simulink model "PHVS_WithACC"  (R2019b)
settings: Solver=VariableStepAuto  StartTime=0.0  StopTime=1.5  FixedStep=0.00001  MinStep=0.0001  RelTol=1e-3
libraries: fl_lib x25, nesl_utility x11, cstblocks x1
settings Model: Creator=se108102  LastModifiedBy=se108102
settings SFSimCC: CustomCodeUndefinedFunction=UseInterfaceOnly

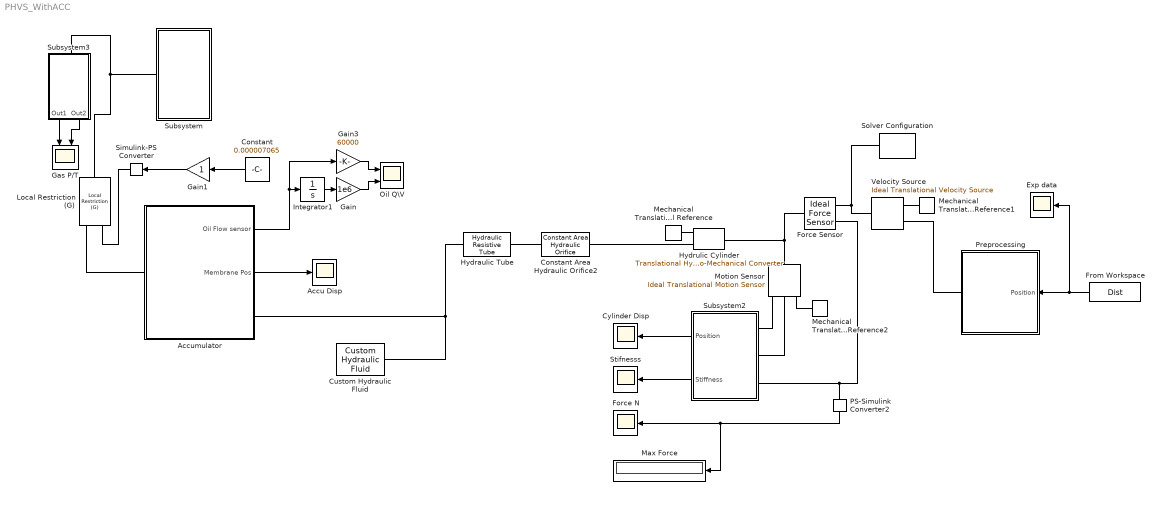
== system PHVS_WithACC ==
  " Force Sensor" : fl_lib/Mechanical/Mechanical Sensors/Ideal Force Sensor
  "Accu Disp " : Scope
  Accumulator : Subsystem
      mask Display: image('ACC.JPG'); % Use "Edit Image" on toolstrip to change.
  Constant : Constant  Value=0.000007065
  Constant Area Hydraulic Orifice2 : fl_lib/Hydraulic/Hydraulic Elements/Constant Area Hydraulic Orifice  area=19.62 mm^2  C_d=.41  lam_spec=1  B_lam=0.999  Re_cr=12  q_specify=off  q_priority=None  q=0.001 m^3/s  q_nominal_specify=off  q_nominal_unit=m^3/s  q_nominal_value=1  p_specify=on  p_priority=None  p=0 Pa  p_nominal_specify=off  p_nominal_unit=Pa  p_nominal_value=1
      settings: SourceProductName=Simscape  SourceProductBaseCode=SS  InternalSimscapePortConfiguration="{\"Bottom\":[],\"Left\":[{\"id\":\"A\",\"label\":\"A\",\"type\":\"foundation.hydraulic.hydraulic\"}],\"Right\":[{\"id\":\"B\",\"label\":\"B\",\"type\":\"foundation.hydraulic.hydraulic\"}],\"Top\":[]}"
  Custom Hydraulic Fluid : fl_lib/Hydraulic/Hydraulic Utilities/Custom Hydraulic Fluid  density=850 kg/m^3  viscosity_kin=18e-6 m^2/s  bulk=0.8e9 Pa  alpha=0.005  range_error=2
      settings: SourceProductName=Simscape  SourceProductBaseCode=SS  InternalSimscapePortConfiguration="{\"Bottom\":[],\"Left\":[],\"Right\":[{\"id\":\"G\",\"label\":\"\",\"type\":\"foundation.hydraulic.hydraulic\"}],\"Top\":[]}"
  Cylinder Disp : Scope
  Exp data : Scope
  Force N : Scope
  From Workspace : FromWorkspace  VariableName=Dist
  Gain : Gain  Gain=1e6
  Gain1 : Gain
  Gain3 : Gain  Gain=60000
  Gas P/T : Scope  NumInputPorts=2
  Hydraulic Tube : fl_lib/Hydraulic/Hydraulic Elements/Hydraulic Resistive Tube  cs_type=1  d_in=10 mm  area=1e-4 m^2  D_h=1.12e-2 m  s_factor=64  length=10 cm  length_ad=1 m  roughness=15e-6 m  Re_lam=2000  Re_turb=4000  q_specify=off  q_priority=None  q=0.001 m^3/s  q_nominal_specify=off  q_nominal_unit=m^3/s  q_nominal_value=1  p_specify=off  p_priority=None  p=0 Pa  p_nominal_specify=off  p_nominal_unit=Pa  p_nominal_value=1
      settings: SourceProductName=Simscape  SourceProductBaseCode=SS  InternalSimscapePortConfiguration="{\"Bottom\":[],\"Left\":[{\"id\":\"A\",\"label\":\"A\",\"type\":\"foundation.hydraulic.hydraulic\"}],\"Right\":[{\"id\":\"B\",\"label\":\"B\",\"type\":\"foundation.hydraulic.hydraulic\"}],\"Top\":[]}"
  Hydrulic Cylinder : fl_lib/Hydraulic/Hydraulic Elements/Translational Hydro-Mechanical Converter  area=12.56 cm^2  or=1  compressibility=0  init_pos=0 m  V_dead=1e-4 m^3  k_sh=1.4  initial_pressure=0 Pa
      settings: SourceProductName=Simscape  SourceProductBaseCode=SS  InternalSimscapePortConfiguration="{\"Bottom\":[],\"Left\":[{\"id\":\"C\",\"label\":\"C\",\"type\":\"foundation.mechanical.translational.translational\"},{\"id\":\"A\",\"label\":\"A\",\"type\":\"foundation.hydraulic.hydraulic\"}],\"Right\":[{\"id\":\"R\",\"label\":\"R\",\"type\":\"foundation.mechanical.translational.translational\"}],\"Top\":[]}"
  Integrator1 : Integrator
  Local Restriction (G) : fl_lib/Gas/Elements/Local Restriction (G)  restriction_type=foundation.enum.restriction_type.variable  restriction_area=1e-3 m^2  min_area=1e-10 m^2  max_area=0.005 m^2  area=0.01 m^2  Cd=0.02  B_lam=0.999
      settings: SourceProductName=Simscape  SourceProductBaseCode=SS  InternalSimscapePortConfiguration="{\"Bottom\":[],\"Left\":[{\"id\":\"A\",\"label\":\"A\",\"type\":\"foundation.gas.gas\"},{\"id\":\"area_in\",\"label\":\"AR\",\"type\":\"input\"}],\"Right\":[{\"id\":\"B\",\"label\":\"B\",\"type\":\"foundation.gas.gas\"}],\"Top\":[]}"
  Max Force : Display
  Mechanical Translational Reference : fl_lib/Mechanical/Translational Elements/Mechanical Translational Reference
  Mechanical Translational Reference1 : fl_lib/Mechanical/Translational Elements/Mechanical Translational Reference
  Mechanical Translational Reference2 : fl_lib/Mechanical/Translational Elements/Mechanical Translational Reference
  Motion Sensor : fl_lib/Mechanical/Mechanical Sensors/Ideal Translational Motion Sensor  offset=0 m
  Oil Q\V : Scope  NumInputPorts=2
  PS-Simulink Converter2 : nesl_utility/PS-Simulink Converter  PhysicalDomain=network_engine_domain  SubClassName=ps_output  LeftPortType=input  RightPortType=output  PseudoPeriodic=off  Frequencies=[]  Unit=N  AffineConversion=off
  "Preprocessing " : Subsystem
      mask Display: image('Icon.png'); % Use "Edit Image" on toolstrip to change.
  Simulink-PS Converter : nesl_utility/Simulink-PS Converter  PhysicalDomain=network_engine_domain  SubClassName=ps_input  LeftPortType=input  RightPortType=output  PseudoPeriodic=off  Frequencies=[]  NoiseDistribution=none  NoiseParameters=[]  Unit=1  AffineConversion=off  FilteringAndDerivatives=provide  SimscapeFilterOrder=1  InputFilterTimeConstant=0.001  UdotUserProvided=0
  Solver Configuration : nesl_utility/Solver Configuration  PhysicalDomain=network_engine_domain  SubClassName=solver  LeftPortType=input  RightPortType=generic  Tones=[]  Harmonics=[]  SimulateNoise=off  Profile=off  UseLocalSampling=off  EnableSwitchedLinearOptims=on  FrequencyDomain=off  UseCCode=off  RelTol=0.001  AbsTol=1e-06  MinStep=1e-09  ToWorkspace=off  RevertToSquareIcSolve=off  NumHomotopyIterations=100  PhasorMode=off  PhasorModeNumHarmonics=1  DoDC=off  ResidualTolerance=1e-09  UseLocalSolver=off  LocalSolverChoice=NE_BACKWARD_EULER_ADVANCER  LocalSolverSampleTime=0.001  DoFixedCost=off  MaxNonlinIter=3  MaxModeIter=2  LinearAlgebra=auto  EquationFormulation=NE_TIME_EF  DelaysMemoryBudget=1024  AutomaticFiltering=on  FilteringTimeConstant=0.001  PartitionStorageMethod=AS_NEEDED  PartitionMemoryBudget=1024  PartitionMethod=ROBUST
  Stifnesss : Scope
  Subsystem : Subsystem
      mask Display: image('Res.png'); % Use "Edit Image" on toolstrip to change.
  Subsystem2 : Subsystem
  Subsystem3 : Subsystem
  Velocity Source : fl_lib/Mechanical/Mechanical Sources/Ideal Translational Velocity Source
  wires:
  Integrator1/1 -> Gain/1
  Accumulator/2(Membrane Pos) -> "Accu Disp "/1
  Accumulator/1(Oil Flow sensor) -> Gain3/1, Integrator1/1
  Subsystem2/1(Position) -> Cylinder Disp/1
  Subsystem2/2(Stiffness) -> Stifnesss/1
  PS-Simulink Converter2/1 -> Max Force/1, Force N/1
  Subsystem3/1(Out1) -> Gas P/T/1
  Subsystem3/2(Out2) -> Gas P/T/2
  From Workspace/1 -> "Preprocessing "/1(Position), Exp data/1
  Gain/1 -> Oil Q\V/2
  Gain3/1 -> Oil Q\V/1
  Constant/1 -> Gain1/1
  Gain1/1 -> Simulink-PS Converter/1
  connections:
  " Force Sensor"/RConn1 -- Velocity Source/LConn1 -- Solver Configuration/RConn1
  Mechanical Translational Reference1/LConn1 -- Velocity Source/RConn2
  Mechanical Translational Reference/LConn1 -- Hydrulic Cylinder/LConn1
  Constant Area Hydraulic Orifice2/RConn1 -- Hydrulic Cylinder/LConn2
  Subsystem3/LConn1 -- Local Restriction (G)/RConn1 -- Subsystem/LConn1
  Hydraulic Tube/LConn1 -- Custom Hydraulic Fluid/RConn1 -- Accumulator/RConn1
  " Force Sensor"/LConn1 -- Motion Sensor/LConn1 -- Hydrulic Cylinder/RConn1
  Subsystem2/LConn3 -- " Force Sensor"/RConn2 -- PS-Simulink Converter2/LConn1
  Motion Sensor/RConn1 -- Mechanical Translational Reference2/LConn1
  Motion Sensor/RConn3 -- Subsystem2/LConn1
  Motion Sensor/RConn2 -- Subsystem2/LConn2
  "Preprocessing "/RConn1 -- Velocity Source/RConn1
  Hydraulic Tube/RConn1 -- Constant Area Hydraulic Orifice2/LConn1
  Local Restriction (G)/LConn1 -- Accumulator/LConn1
  Local Restriction (G)/LConn2 -- Simulink-PS Converter/RConn1

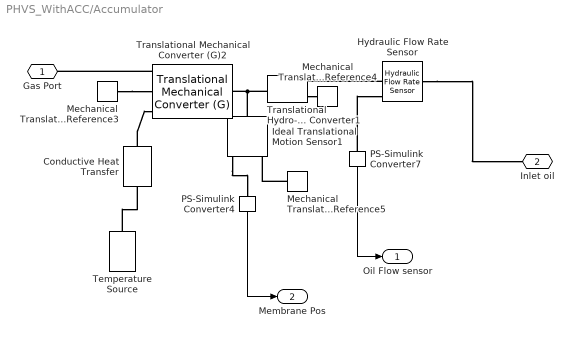
== system PHVS_WithACC/Accumulator ==
  Conductive Heat Transfer : fl_lib/Thermal/Thermal Elements/Conductive Heat Transfer  area=60 cm^2  thickness=1 mm  th_cond=205 W/(m*K)  T_specify=on  T_priority=High  T=0 degC  T_nominal_specify=off  T_nominal_unit=K  T_nominal_value=1  Q_specify=off  Q_priority=High  Q=0 W  Q_nominal_specify=off  Q_nominal_unit=W  Q_nominal_value=1
      settings: SourceProductName=Simscape
  Hydraulic Flow Rate Sensor : fl_lib/Hydraulic/Hydraulic Sensors/Hydraulic Flow Rate Sensor
      settings: SourceProductName=Simscape
  Ideal Translational Motion Sensor1 : fl_lib/Mechanical/Mechanical Sensors/Ideal Translational Motion Sensor  offset=0 m
  Mechanical Translational Reference3 : fl_lib/Mechanical/Translational Elements/Mechanical Translational Reference
  Mechanical Translational Reference4 : fl_lib/Mechanical/Translational Elements/Mechanical Translational Reference
  Mechanical Translational Reference5 : fl_lib/Mechanical/Translational Elements/Mechanical Translational Reference
  PS-Simulink Converter4 : nesl_utility/PS-Simulink Converter  PhysicalDomain=network_engine_domain  SubClassName=ps_output  LeftPortType=input  RightPortType=output  PseudoPeriodic=off  Frequencies=[]  Unit=m  AffineConversion=off
  PS-Simulink Converter7 : nesl_utility/PS-Simulink Converter  PhysicalDomain=network_engine_domain  SubClassName=ps_output  LeftPortType=input  RightPortType=output  PseudoPeriodic=off  Frequencies=[]  Unit=m^3/s  AffineConversion=off
  Temperature Source : fl_lib/Thermal/Thermal Sources/Temperature Source  temperature=25 degC
      settings: SourceProductName=Simscape
  Translational Hydro-Mechanical Converter1 : fl_lib/Hydraulic/Hydraulic Elements/Translational Hydro-Mechanical Converter  area=12.56 cm^2  or=2  compressibility=0  init_pos=0 m  V_dead=1e-4 m^3  k_sh=1.4  initial_pressure=0 Pa
      settings: SourceProductName=Simscape  SourceProductBaseCode=SS  InternalSimscapePortConfiguration="{\"Bottom\":[],\"Left\":[{\"id\":\"C\",\"label\":\"C\",\"type\":\"foundation.mechanical.translational.translational\"},{\"id\":\"A\",\"label\":\"A\",\"type\":\"foundation.hydraulic.hydraulic\"}],\"Right\":[{\"id\":\"R\",\"label\":\"R\",\"type\":\"foundation.mechanical.translational.translational\"}],\"Top\":[]}"
  Translational Mechanical Converter (G)2 : fl_lib/Gas/Elements/Translational Mechanical Converter (G)  mech_orientation=simscape.enum.posneg.positive  interface_area=12.56 cm^2  length_init=18 mm  dead_volume=1 cm^3  area_A=7.06 mm^2  environment_spec=foundation.enum.pressure_spec.atmospheric  environment_pressure=1 bar  p_I_specify=off  p_I_priority=Low  p_I=1.3 bar  p_I_nominal_specify=off  p_I_nominal_unit=MPa  p_I_nominal_value=1  T_I_specify=on  T_I_priority=High  T_I=25 degC  T_I_nominal_specify=off  T_I_nominal_unit=K  T_I_nominal_value=1  rho_converter_specify=off  rho_converter_priority=None  rho_converter=1.2 kg/m^3  rho_converter_nominal_specify=off  rho_converter_nominal_unit=kg/m^3  rho_converter_nominal_value=1
      settings: SourceProductName=Simscape  SourceProductBaseCode=SS  InternalSimscapePortConfiguration="{\"Bottom\":[],\"Left\":[{\"id\":\"A\",\"label\":\"A\",\"type\":\"foundation.gas.gas\"},{\"id\":\"C\",\"label\":\"C\",\"type\":\"foundation.mechanical.translational.translational\"},{\"id\":\"H\",\"label\":\"H\",\"type\":\"foundation.thermal.thermal\"}],\"Right\":[{\"id\":\"R\",\"label\":\"R\",\"type\":\"foundation.mechanical.translational.translational\"}],\"Top\":[]}"
  Gas Port : PMIOPort  Side=Left
  Inlet oil : PMIOPort  Port=2  Side=Right
  Oil Flow sensor : Outport
  Membrane Pos : Outport  Port=2
  wires:
  PS-Simulink Converter4/1 -> Membrane Pos/1
  PS-Simulink Converter7/1 -> Oil Flow sensor/1
  connections:
  Translational Hydro-Mechanical Converter1/LConn1 -- Mechanical Translational Reference4/LConn1
  Mechanical Translational Reference3/LConn1 -- Translational Mechanical Converter (G)2/LConn2
  Temperature Source/LConn1 -- Conductive Heat Transfer/RConn1
  Translational Hydro-Mechanical Converter1/RConn1 -- Ideal Translational Motion Sensor1/LConn1 -- Translational Mechanical Converter (G)2/RConn1
  Conductive Heat Transfer/LConn1 -- Translational Mechanical Converter (G)2/LConn3
  Ideal Translational Motion Sensor1/RConn3 -- PS-Simulink Converter4/LConn1
  PS-Simulink Converter7/LConn1 -- Hydraulic Flow Rate Sensor/RConn1
  Mechanical Translational Reference5/LConn1 -- Ideal Translational Motion Sensor1/RConn1
  Hydraulic Flow Rate Sensor/LConn1 -- Inlet oil/RConn1
  Hydraulic Flow Rate Sensor/RConn2 -- Translational Hydro-Mechanical Converter1/LConn2
  Translational Mechanical Converter (G)2/LConn1 -- Gas Port/RConn1

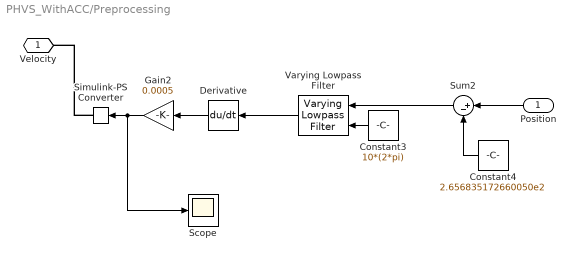
== system PHVS_WithACC/Preprocessing  ==
  Position : Inport
  Constant3 : Constant  Value=10*(2*pi)
  Constant4 : Constant  Value=2.656835172660050e2
  Derivative : Derivative
  Gain2 : Gain  Gain=0.0005
  Scope : Scope
  Simulink-PS Converter : nesl_utility/Simulink-PS Converter  PhysicalDomain=network_engine_domain  SubClassName=ps_input  LeftPortType=input  RightPortType=output  PseudoPeriodic=off  Frequencies=[]  NoiseDistribution=none  NoiseParameters=[]  Unit=1  AffineConversion=off  FilteringAndDerivatives=provide  SimscapeFilterOrder=1  InputFilterTimeConstant=0.001  UdotUserProvided=0
  Sum2 : Sum  Inputs=|+-
  Varying Lowpass Filter : cstblocks/Linear Parameter Varying/Varying Lowpass Filter  N=10
      settings: SourceProductName=Control System Toolbox
  Velocity : PMIOPort  Side=Right
  wires:
  Sum2/1 -> Varying Lowpass Filter/1
  Varying Lowpass Filter/1 -> Derivative/1
  Constant4/1 -> Sum2/2
  Gain2/1 -> Scope/1, Simulink-PS Converter/1
  Constant3/1 -> Varying Lowpass Filter/2
  Derivative/1 -> Gain2/1
  Position/1 -> Sum2/1
  connections:
  Simulink-PS Converter/RConn1 -- Velocity/RConn1

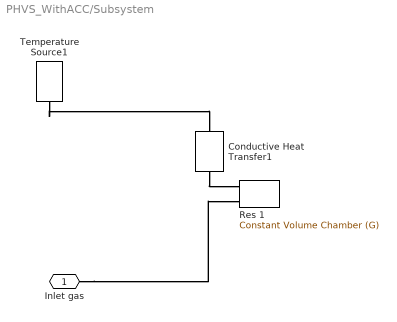
== system PHVS_WithACC/Subsystem ==
  Conductive Heat Transfer1 : fl_lib/Thermal/Thermal Elements/Conductive Heat Transfer  area=12 cm^2  thickness=2.5 mm  th_cond=50 W/(m*K)  T_specify=off  T_priority=High  T=0 degC  T_nominal_specify=off  T_nominal_unit=K  T_nominal_value=1  Q_specify=off  Q_priority=None  Q=0 W  Q_nominal_specify=off  Q_nominal_unit=W  Q_nominal_value=1
      settings: SourceProductName=Simscape
  "Res 1 " : fl_lib/Gas/Elements/Constant Volume Chamber (G)  volume=1 cm^3  num_ports=foundation.enum.num_ports.one  area_A=7.5 mm^2  area_B=0.01 m^2  area_C=0.01 m^2  area_D=0.01 m^2  p_I_specify=off  p_I_priority=None  p_I=1.3 bar  p_I_nominal_specify=off  p_I_nominal_unit=MPa  p_I_nominal_value=1  T_I_specify=on  T_I_priority=Low  T_I=25 degC  T_I_nominal_specify=off  T_I_nominal_unit=K  T_I_nominal_value=1  rho_chamber_specify=off  rho_chamber_priority=None  rho_chamber=1.2 kg/m^3  rho_chamber_nominal_specify=off  rho_chamber_nominal_unit=kg/m^3  rho_chamber_nominal_value=1
      settings: SourceProductName=Simscape  SourceProductBaseCode=SS  InternalSimscapePortConfiguration="{\"Bottom\":[],\"Left\":[{\"id\":\"A\",\"label\":\"A\",\"type\":\"foundation.gas.gas\"},{\"id\":\"H\",\"label\":\"H\",\"type\":\"foundation.thermal.thermal\"}],\"Right\":[],\"Top\":[]}"
  Temperature Source1 : fl_lib/Thermal/Thermal Sources/Temperature Source  temperature=25 degC
      settings: SourceProductName=Simscape
  Inlet gas : PMIOPort  Side=Left
  connections:
  Temperature Source1/LConn1 -- Conductive Heat Transfer1/RConn1
  Conductive Heat Transfer1/LConn1 -- "Res 1 "/LConn2
  Inlet gas/RConn1 -- "Res 1 "/LConn1

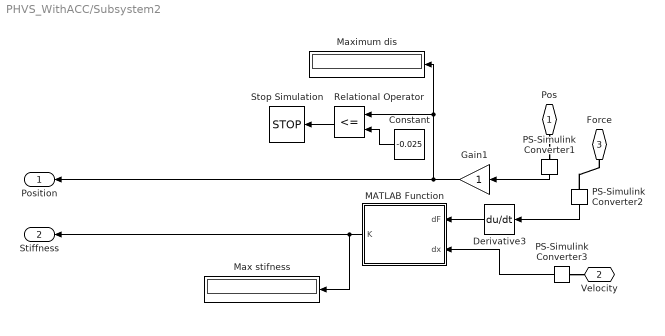
== system PHVS_WithACC/Subsystem2 ==
  Constant : Constant  Value=-0.025
  Derivative3 : Derivative
  Gain1 : Gain
  MATLAB Function : MATLAB Function  TreatAsAtomicUnit=on
  Max stifness : Display
  Maximum dis : Display
  PS-Simulink Converter1 : nesl_utility/PS-Simulink Converter  PhysicalDomain=network_engine_domain  SubClassName=ps_output  LeftPortType=input  RightPortType=output  PseudoPeriodic=off  Frequencies=[]  Unit=m  AffineConversion=off
  PS-Simulink Converter2 : nesl_utility/PS-Simulink Converter  PhysicalDomain=network_engine_domain  SubClassName=ps_output  LeftPortType=input  RightPortType=output  PseudoPeriodic=off  Frequencies=[]  Unit=N  AffineConversion=off
  PS-Simulink Converter3 : nesl_utility/PS-Simulink Converter  PhysicalDomain=network_engine_domain  SubClassName=ps_output  LeftPortType=input  RightPortType=output  PseudoPeriodic=off  Frequencies=[]  Unit=m/s  AffineConversion=off
  Relational Operator : RelationalOperator  Operator=<=  OutDataTypeStr=boolean  RndMeth=Simplest
  Stop Simulation : Stop
  Pos : PMIOPort  Side=Left
  Velocity : PMIOPort  Port=2  Side=Left
  Force : PMIOPort  Port=3  Side=Left
  Position : Outport
  Stiffness : Outport  Port=2
  wires:
  PS-Simulink Converter1/1 -> Gain1/1
  PS-Simulink Converter2/1 -> Derivative3/1
  MATLAB Function/1(K) -> Max stifness/1, Stiffness/1
  Constant/1 -> Relational Operator/2
  Derivative3/1 -> MATLAB Function/1(dF)
  Gain1/1 -> Position/1, Relational Operator/1, Maximum dis/1
  Relational Operator/1 -> Stop Simulation/1
  PS-Simulink Converter3/1 -> MATLAB Function/2(dx)
  connections:
  PS-Simulink Converter2/LConn1 -- Force/RConn1
  Pos/RConn1 -- PS-Simulink Converter1/LConn1
  PS-Simulink Converter3/LConn1 -- Velocity/RConn1

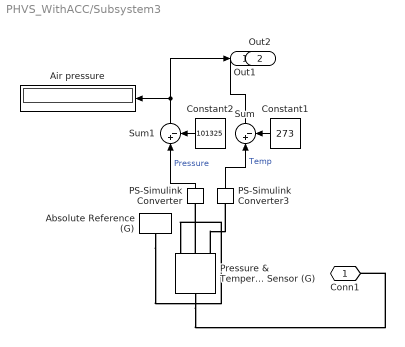
== system PHVS_WithACC/Subsystem3 ==
  Absolute Reference (G) : fl_lib/Gas/Elements/Absolute Reference (G)
      settings: SourceProductName=Simscape  SourceProductBaseCode=SS  InternalSimscapePortConfiguration="{\"Bottom\":[],\"Left\":[{\"id\":\"A\",\"label\":\"\",\"type\":\"foundation.gas.gas\"}],\"Right\":[],\"Top\":[]}"
  Air pressure : Display
  Constant1 : Constant  Value=273
  Constant2 : Constant  Value=101325
  PS-Simulink Converter : nesl_utility/PS-Simulink Converter  PhysicalDomain=network_engine_domain  SubClassName=ps_output  LeftPortType=input  RightPortType=output  PseudoPeriodic=off  Frequencies=[]  Unit=Pa  AffineConversion=off
  PS-Simulink Converter3 : nesl_utility/PS-Simulink Converter  PhysicalDomain=network_engine_domain  SubClassName=ps_output  LeftPortType=input  RightPortType=output  PseudoPeriodic=off  Frequencies=[]  Unit=K  AffineConversion=off
  Pressure & Temperature Sensor (G) : fl_lib/Gas/Sensors/Pressure & Temperature Sensor (G)
      settings: SourceProductName=Simscape  SourceProductBaseCode=SS  InternalSimscapePortConfiguration="{\"Bottom\":[],\"Left\":[{\"id\":\"A\",\"label\":\"A\",\"type\":\"foundation.gas.gas\"}],\"Right\":[{\"id\":\"B\",\"label\":\"B\",\"type\":\"foundation.gas.gas\"},{\"id\":\"P\",\"label\":\"P\",\"type\":\"output\"},{\"id\":\"T\",\"label\":\"T\",\"type\":\"output\"}],\"Top\":[]}"
  Sum : Sum  Inputs=|+-
  Sum1 : Sum  Inputs=|+-
  Conn1 : PMIOPort  Side=Left
  Out1 : Outport
  Out2 : Outport  Port=2
  wires:
  PS-Simulink Converter3/1 -> Sum/1  "Temp"
  Constant2/1 -> Sum1/2
  Sum1/1 -> Out1/1, Air pressure/1
  PS-Simulink Converter/1 -> Sum1/1  "Pressure"
  Constant1/1 -> Sum/2
  Sum/1 -> Out2/1
  connections:
  Absolute Reference (G)/LConn1 -- Pressure & Temperature Sensor (G)/RConn1
  Pressure & Temperature Sensor (G)/RConn3 -- PS-Simulink Converter3/LConn1
  Pressure & Temperature Sensor (G)/RConn2 -- PS-Simulink Converter/LConn1
  Pressure & Temperature Sensor (G)/LConn1 -- Conn1/RConn1

== matlab function PHVS_WithACC/Subsystem2/MATLAB Function ==
  data: dF input; K output; dx input
function K = fcn(dF,dx)
if dF<0
    dF=0;
end
dx=-0.03;
K = -1*dF/dx;
